simulink model "close_loop_"  (R2018a)
settings: Solver=ode4  StartTime=0.0  StopTime=4  FixedStep=0.001  RelTol=1e-3
undefined symbols (not defined in the file): Km, Kp, Wm, Zm
settings Model: Creator=msi  LastModifiedBy=xde12

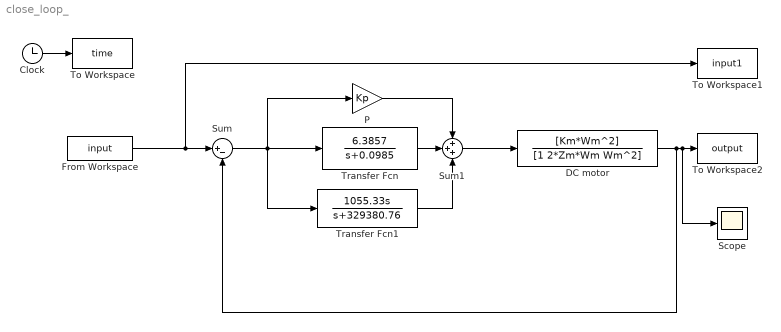
== system close_loop_ ==
  Clock : Clock
  DC motor : TransferFcn  Numerator=[Km*Wm^2]  Denominator=[1 2*Zm*Wm Wm^2]
  From Workspace : FromWorkspace  VariableName=input  SampleTime=0
  P : Gain  Gain=Kp
  Scope : Scope
  Sum : Sum  Inputs=|+-
  Sum1 : Sum  Inputs=+++
  To Workspace : ToWorkspace  VariableName=time  SampleTime=-1
  To Workspace1 : ToWorkspace  VariableName=input1  SampleTime=-1
  To Workspace2 : ToWorkspace  VariableName=output  SampleTime=-1
  Transfer Fcn : TransferFcn  Numerator=[6.3857]  Denominator=[1 0.0985]
  Transfer Fcn1 : TransferFcn  Numerator=[1055.33 0 ]  Denominator=[1 329380.76]
  wires:
  Sum/1 -> Transfer Fcn1/1, Transfer Fcn/1, P/1
  P/1 -> Sum1/1
  Sum1/1 -> DC motor/1
  Clock/1 -> To Workspace/1
  From Workspace/1 -> Sum/1, To Workspace1/1
  Transfer Fcn/1 -> Sum1/2
  Transfer Fcn1/1 -> Sum1/3
  DC motor/1 -> Scope/1, To Workspace2/1, Sum/2
